simulink model "state_controller"  (R2015b)
settings: Solver=FixedStepDiscrete  StartTime=0.0  StopTime=0  FixedStep=Ts  RelTol=1e-3
values from neighbouring files (symbols this model uses):
  ground_data = zeros(2, 5)    [BipedVisualization.m]    (also in Planner.m; biped_setup.m = [ground_x, ground_y, ground_stiffness, ground_damping, groun)
  params = zeros(11, 1)    [DoubleSupportController.m]    (also in FlightController.m; LegController.m; PlanarBipedController.m = zeros(12, 1); Sequencing.m)
  Ts = 1e-3    (= 0.001)    [BipedController.m]    (also in LegController.m; Planner.m = 0.1; Sequencing.m; StateEstimator.m)
settings Model: Creator=robots  LastModifiedBy=robot

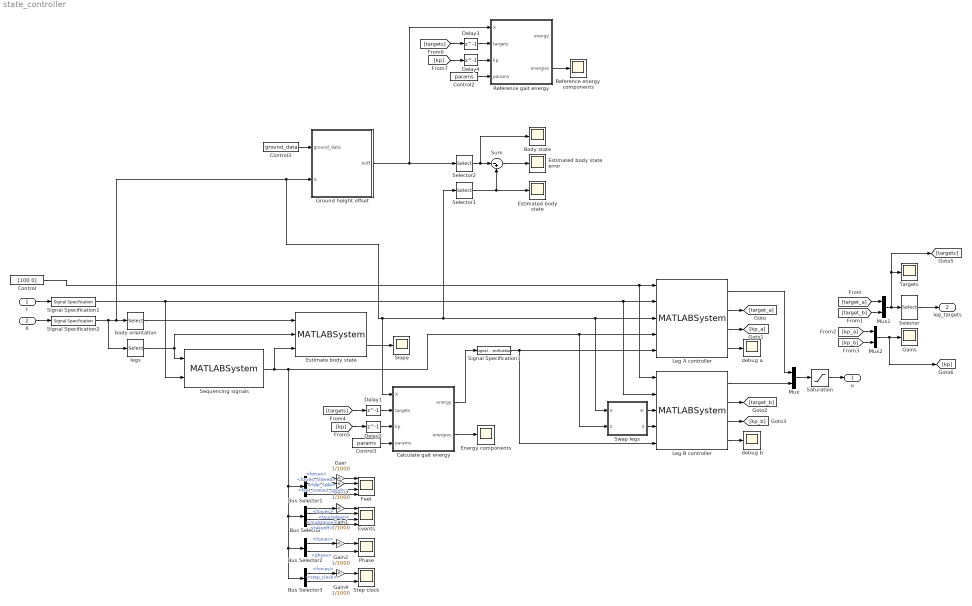
== system state_controller ==
  t : Inport
  X : Inport  Port=2
  Body state : Scope
  Bus Selector : BusSelector  OutputSignals=forces,touchdown,midstance,takeoff
  Bus Selector1 : BusSelector  OutputSignals=forces,forces_filtered,feet_fade,feet_contact_good
  Bus Selector2 : BusSelector  OutputSignals=forces,phase
  Bus Selector3 : BusSelector  OutputSignals=forces,step_clock
  Calculate gait energy : MATLAB Function  TreatAsAtomicUnit=on
  Control : Constant  Value=[100 0]
  Control1 : Constant  Value=params
  Control2 : Constant  Value=params
  Control3 : Constant  Value=ground_data
  Delay{1..4} (4 alike) : Delay  DelayLength=1  InitialCondition=0
  Energy components : Scope
  Estimate body state : MATLABSystem  System=StateEstimator  Ts=Ts  params=params  SimulateUsing=Code generation
      mask Type: StateEstimator
      mask Display:
      | disp('StateEstimator');
      | port_label('input',1,'orientation');
      | port_label('input',2,'legs');
      | port_label('input',3,'signals');
      | port_label('output',1,'X');
      | port_label('output',2,'slope');
  Estimated body state : Scope
  Estimated body state error : Scope
  Events : Scope  NumInputPorts=4
  Feet : Scope  NumInputPorts=4
  Gain{,1..4} (5 alike) : Gain  Gain=1/1000
  Gains : Scope
  Ground height offset : MATLAB Function  TreatAsAtomicUnit=on
  Leg A controller : MATLABSystem  System=LegController  Ts=Ts  params=params  kp_ground=kp_ground  kd_ground=kd_ground  kp_air=kp_air  kd_air=kd_air  leq_neutral=1  step_period=step_period  SimulateUsing=Code generation
      mask Type: LegController
      mask Display:
      | disp('LegController');
      | port_label('input',1,'control');
      | port_label('input',2,'t');
      | port_label('input',3,'X');
      | port_label('input',4,'signals');
      | port_label('input',5,'energy');
      | port_label('output',1,'u');
      | port_label('output',2,'target');
      | port_label('output',3,'kp');
      | port_label('output',4,'debug');
  Leg B controller : MATLABSystem  System=LegController  Ts=Ts  params=params  kp_ground=kp_ground  kd_ground=kd_ground  kp_air=kp_air  kd_air=kd_air  leq_neutral=1  step_period=step_period  SimulateUsing=Code generation
      mask Type: LegController
      mask Display:
      | disp('LegController');
      | port_label('input',1,'control');
      | port_label('input',2,'t');
      | port_label('input',3,'X');
      | port_label('input',4,'signals');
      | port_label('input',5,'energy');
      | port_label('output',1,'u');
      | port_label('output',2,'target');
      | port_label('output',3,'kp');
      | port_label('output',4,'debug');
  Mux : Mux  Inputs=2
  Mux1 : Mux  Inputs=2
  Mux2 : Mux  Inputs=2
  Phase : Scope  NumInputPorts=2
  Reference energy components : Scope
  Reference gait energy : MATLAB Function  TreatAsAtomicUnit=on
  Saturation : Saturate  UpperLimit=[3e3 3e1 3e3 3e1]'  LowerLimit=-[3e3 3e1 3e3 3e1]'
  Selector : Selector  InputPortWidth=6  IndexOptions=Index vector (dialog)  Indices=[1 2 4 5]  OutputSizes=1
  Selector1 : Selector  InputPortWidth=18  IndexOptions=Index vector (dialog)  Indices=[1:4]  OutputSizes=1
  Selector2 : Selector  InputPortWidth=18  IndexOptions=Index vector (dialog)  Indices=[1:4]  OutputSizes=1
  Sequencing signals : MATLABSystem  System=Sequencing  Ts=Ts  params=params  filter_constant=0.04  step_period=step_period  OutputBusName=sequencing_signal_bus  SimulateUsing=Code generation
      mask Type: Sequencing
      mask Display:
      | disp('Sequencing');
      | port_label('input',1,'legs');
      | port_label('input',2,'t');
      | port_label('output',1,'signals');
  Signal Specification1 : SignalSpecification  OutDataTypeStr=double  Dimensions=[1 1]
  Signal Specification2 : SignalSpecification  OutDataTypeStr=double  Dimensions=[18 1]
  Signal Specification3 : SignalSpecification  OutDataTypeStr=double  Dimensions=[1 1]
  Slope : Scope
  Step clock : Scope  NumInputPorts=2
  Sum : Sum  Inputs=|-+
  Swap legs : Subsystem
  Targets : Scope
  body orientation : Selector  InputPortWidth=18  IndexOptions=Index vector (dialog)  Indices=[5:6]  OutputSizes=1
  debug a : Scope
  debug b : Scope
  legs : Selector  InputPortWidth=18  IndexOptions=Index vector (dialog)  Indices=[7:18]  OutputSizes=1
  u : Outport
  leg_targets : Outport  Port=2
  wires:
  X/1 -> Signal Specification2/1
  Control/1 -> Leg B controller/1, Leg A controller/1
  t/1 -> Signal Specification1/1
  Leg A controller/1 -> Mux/1
  Leg B controller/1 -> Mux/2
  Mux/1 -> Saturation/1
  Leg A controller/4 -> debug a/1
  Leg A controller/2 -> [target_a]
  Leg B controller/2 -> [target_b]
  Leg A controller/3 -> [kp_a]
  Leg B controller/3 -> [kp_b]
  Mux2/1 -> Gains/1, [kp]
  Saturation/1 -> u/1
  [target_a] -> Mux1/1
  [target_b] -> Mux1/2
  [kp_a] -> Mux2/1
  [kp_b] -> Mux2/2
  Selector/1 -> leg_targets/1
  Swap legs/1(X') -> Leg B controller/3
  Leg B controller/4 -> debug b/1
  Mux1/1 -> [targets], Targets/1, Selector/1
  Control1/1 -> Calculate gait energy/4(params)
  Calculate gait energy/1(energy) -> Signal Specification3/1
  Calculate gait energy/2(energies) -> Energy components/1
  [targets] -> Delay1/1
  [kp] -> Delay2/1
  Signal Specification1/1 -> Sequencing signals/2, Leg A controller/2, Leg B controller/2
  legs/1 -> Sequencing signals/1, Estimate body state/2
  Delay2/1 -> Calculate gait energy/3(kp)
  Delay1/1 -> Calculate gait energy/2(targets)
  Signal Specification3/1 -> Leg B controller/5, Leg A controller/5
  body orientation/1 -> Estimate body state/1
  Sequencing signals/1 -> Leg A controller/4, Swap legs/2(signals), Bus Selector1/1, Bus Selector3/1, Bus Selector2/1, Bus Selector/1, Estimate body state/3
  Estimate body state/2 -> Slope/1
  Swap legs/2(signals') -> Leg B controller/4
  [kp] -> Delay4/1
  Control3/1 -> Ground height offset/1(ground_data)
  [targets] -> Delay3/1
  Reference gait energy/2(energies) -> Reference energy components/1
  Delay4/1 -> Reference gait energy/3(kp)
  Ground height offset/1(Xoff) -> Reference gait energy/1(X), Selector2/1
  Control2/1 -> Reference gait energy/4(params)
  Delay3/1 -> Reference gait energy/2(targets)
  Sum/1 -> Estimated body state error/1
  Selector2/1 -> Body state/1, Sum/1
  Selector1/1 -> Sum/2, Estimated body state/1
  Signal Specification2/1 -> legs/1, Calculate gait energy/1(X), Swap legs/1(X), Leg A controller/3, Selector1/1, Ground height offset/2(X), body orientation/1
  Bus Selector1/1 -> Gain/1  "<forces>"
  Bus Selector1/3 -> Feet/3  "<feet_fade>"
  Bus Selector1/4 -> Feet/4  "<feet_contact_good>"
  Bus Selector/1 -> Gain1/1  "<forces>"
  Bus Selector/2 -> Events/2  "<touchdown>"
  Bus Selector/3 -> Events/3  "<midstance>"
  Bus Selector/4 -> Events/4  "<takeoff>"
  Bus Selector2/1 -> Gain2/1  "<forces>"
  Bus Selector2/2 -> Phase/2  "<phase>"
  Gain/1 -> Feet/1
  Gain1/1 -> Events/1
  Gain2/1 -> Phase/1
  Bus Selector1/2 -> Gain3/1  "<forces_filtered>"
  Gain3/1 -> Feet/2
  Gain4/1 -> Step clock/1
  Bus Selector3/1 -> Gain4/1  "<forces>"
  Bus Selector3/2 -> Step clock/2  "<step_clock>"

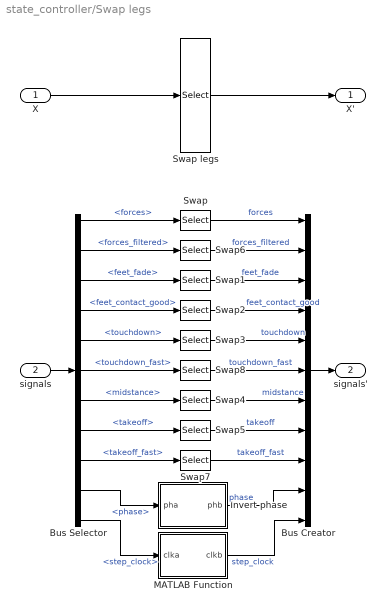
== system state_controller/Swap legs ==
  X : Inport
  signals : Inport  Port=2
  Bus Creator : BusCreator  Inputs='forces','forces_filtered','feet_fade','feet_contact_good','touchdown','touchdown_fast','midstance','takeoff','takeoff_fast','phase','step_clock'  OutDataTypeStr=Bus: sequencing_signal_bus  NonVirtualBus=on
  Bus Selector : BusSelector  OutputSignals=forces,forces_filtered,feet_fade,feet_contact_good,touchdown,touchdown_fast,midstance,takeoff,takeoff_fast,phase,step_clock
  Invert phase : MATLAB Function  TreatAsAtomicUnit=on
  MATLAB Function : MATLAB Function  TreatAsAtomicUnit=on
  Swap{,1..8} (9 alike) : Selector  InputPortWidth=2  IndexOptions=Index vector (dialog)  Indices=[2 1]  OutputSizes=1
  Swap legs : Selector  InputPortWidth=18  IndexOptions=Index vector (dialog)  Indices=[1:6 13:18 7:12]  OutputSizes=1
  X' : Outport
  signals' : Outport  Port=2
  wires:
  Swap legs/1 -> X'/1
  X/1 -> Swap legs/1
  signals/1 -> Bus Selector/1
  Bus Creator/1 -> signals'/1
  Bus Selector/1 -> Swap/1  "<forces>"
  Bus Selector/3 -> Swap1/1  "<feet_fade>"
  Bus Selector/4 -> Swap2/1  "<feet_contact_good>"
  Bus Selector/5 -> Swap3/1  "<touchdown>"
  Bus Selector/7 -> Swap4/1  "<midstance>"
  Bus Selector/8 -> Swap5/1  "<takeoff>"
  Swap/1 -> Bus Creator/1  "forces"
  Swap1/1 -> Bus Creator/3  "feet_fade"
  Swap2/1 -> Bus Creator/4  "feet_contact_good"
  Swap3/1 -> Bus Creator/5  "touchdown"
  Swap4/1 -> Bus Creator/7  "midstance"
  Swap5/1 -> Bus Creator/8  "takeoff"
  Bus Selector/10 -> Invert phase/1(pha)  "<phase>"
  Invert phase/1(phb) -> Bus Creator/10  "phase"
  Bus Selector/2 -> Swap6/1  "<forces_filtered>"
  Swap6/1 -> Bus Creator/2  "forces_filtered"
  Bus Selector/6 -> Swap8/1  "<touchdown_fast>"
  Swap8/1 -> Bus Creator/6  "touchdown_fast"
  Bus Selector/9 -> Swap7/1  "<takeoff_fast>"
  Swap7/1 -> Bus Creator/9  "takeoff_fast"
  Bus Selector/11 -> MATLAB Function/1(clka)  "<step_clock>"
  MATLAB Function/1(clkb) -> Bus Creator/11  "step_clock"

== matlab function state_controller/Swap legs/MATLAB Function ==
  data: clka input; clkb output
function clkb = invert_clock(clka) %#codegen

clkb = mod(clka + 0.5, 1);

== matlab function state_controller/Reference gait energy ==
  data: X input; energy output; targets input; kp input; params input; energies output
function [energy, energies] = gait_energy(X, targets, kp, params) %#codegen

[energy, energies] = gait_energy(X, targets, kp, params);

== matlab function state_controller/Swap legs/Invert phase ==
  data: pha input; phb output
function phb = invert_phase(pha) %#codegen

phb = [-pha(1); mod(pha(2) + 2, 4)];

== matlab function state_controller/Ground height offset ==
  data: ground_data input; X input; Xoff output
function Xoff = ground_height_offset(ground_data, X) %#codegen

% Find ground height at body x
[~, yi, ~] = linexpoly([X(1); X(1)], X(3) + [-1e3; 1e3], ground_data(:, 1), ground_data(:, 2));

if ~isempty(yi)
    h = max(yi);
else
    h = 0;
end

% Subtract ground height from absolute y
Xoff = X;
Xoff(3) = Xoff(3) - h;


function [xi, yi, ii] = linexpoly(x1, y1, x2, y2)
% Customized implementation of polyxpoly for codegen
dx1 = x1(2) - x1(1);
dy1 = y1(2) - y1(1);
dx2 = x2(2:end) - x2(1:end-1);
dy2 = y2(2:end) - y2(1:end-1);
dx12 = x1(1) - x2(1:end-1);
dy12 = y1(1) - y2(1:end-1);

num = dx2.*dy12 - dy2.*dx12;
den = dy2.*dx1 - dx2.*dy1;

sa = num./den;
sb = (dx12 + sa.*dx1)./dx2;

ii = find(den ~= 0 & sa >= 0 & sa < 1 & sb >= 0 & sb < 1);
xi = x1(1) + sa(ii).*dx1;
yi = y1(1) + sa(ii).*dy1;

== matlab function state_controller/Calculate gait energy ==
  data: X input; energy output; targets input; kp input; params input; energies output
function [energy, energies] = gait_energy(X, targets, kp, params) %#codegen

[energy, energies] = gait_energy(X, targets, kp, params);
